simulink library "Collector_Unglazed"  (R2018b)
settings: Solver=ode45  StartTime=0.0  StopTime=10.0  RelTol=1e-3  EnableMultiTasking=on
undefined symbols (not defined in the file): Acol, path_carnot, Qdot, THBin, THBout
libraries: carnot x5
settings Model: Creator=bernd.hafner  LastModifiedBy=P41573
settings DataIOCC: LimitDataPoints=on  SaveFormat=Array  SignalLoggingSaveFormat=ModelDataLogs
settings OptimizationCC: ExpressionDepthLimit=2147483647  LifeSpan=inf
settings DebuggingCC: UnderspecifiedInitializationDetection=Classic  MergeDetectMultiDrivingBlocksExec=none  SolverPrmCheckMsg=warning  FcnCallInpInsideContextMsg=warning  StateNameClashWarn=warning  SFUnexpectedBacktrackingDiag=warning  SFNoUnconditionalDefaultTransitionDiag=warning  SFExecutionAtInitializationDiag=none
settings HardwareCC: ProdBitPerPointer=32  ProdBitPerSizeT=32  ProdBitPerPtrDiffT=32  ProdLargestAtomicFloat=None  ProdIntDivRoundTo=Undefined  ProdEndianess=Unspecified  ProdWordSize=32  ProdHWDeviceType=32-bit Generic
settings ModelReferenceCC: PropagateSignalLabelsOutOfModel=off
settings SFSimCC: SimUseLocalCustomCode=off
settings RTWCC: RTWUseLocalCustomCode=off
settings CodeAppCC: StateflowObjectComments=on
settings GRTTargetCC: TargetLangStandard=C89/C90 (ANSI)  GeneratePreprocessorConditionals=Disable all  CombineOutputUpdateFcns=off  GRTInterface=on
settings ConfigComp: CovMetricSettings=dw  CovHtmlReporting=on  CovSaveCumulativeToWorkspaceVar=on  CovSaveSingleToWorkspaceVar=on  CovExternalEMLEnable=off

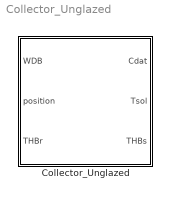
== system Collector_Unglazed ==
  Collector_Unglazed : Subsystem  mask(Unglazed solar thermal collector){tini=0.1, Ncollector=1, PathName=fullfile(path_carnot('libsl'), 'Source', 'Solar_Thermal', 'Collector_Unglazed', 'parameter_set'), FileName='DefaultCollectorUnglazed.mat', userPath=off, userParam=off, acol=2.544, len=2.1, nodes=10, fta=0.9, eps=0.9, u0l=40, u0c=1, u0g=40, u1l=8, u1c=1, u1g=8, u1e=0.01, hi=200, capa=5000, capf=4000, SensorTimeConstant=10, dplin=5504.4, dpqua=6222.096}
      mask prompts: tini "Initial temperature [°C]"; Ncollector "Number of collectors in parallel"; PathName "Path"; FileName "Parameter set"; userPath "Edit path and name of parameter set"; userParam "User defined parameters"; acol "Collector surface (aperture) in [m²]"; len "Length between inlet and outlet [m]"; nodes "Number of nodes (>=2)"; fta "Absorption coefficient of the absorber [-]"; eps "Thermal emissivity of the absorber (0..1)"; u0l "U0L heat transfer for losses [W/(m²*K)]"; u0c "U0C heat transfer for condensation [W/(m²*K)]"; u0g "U0G heat transfer for gains [W/(m²*K)]"; u1l "U1L wind dependent heat transfer for losses [W/(m²*K*m/s)]"; u1c "U1C wind dependent heat transfer for condensation [W/(m²*K*m/s)]"; u1g "U1G wind dependent heat transfer for gains [W/(m²*K*m/s)]"; u1e "U1E wind dependancy of optical efficiency in W/(m²*m/s)"; hi "HI heat transfer between collector and tube [W/(m²*K)]"; capa "Effective heat capacity of absorber [J/(m²*K)]"; capf "Effective heat capacity of fluid [J/(m²*K)]"; SensorTimeConstant "Time constant of temperature sensor [s]"; dplin "Linear pressure drop in Pa/(kg/s)"; dpqua "Quadratic pressure drop in Pa/(kg/s)²"
      mask help:
      | 2xN node model for an unglazed solar thermal collectors including condensation effects for temperatures below dewpoint.
      | c_abs*dTp/dt=qdot_solar-qdot_conv_gain-qdot_conv_loss-qdot_cond -qdot_sky-qdot_fluid
      | qdot_solar = absorbed_solar_radiation - U1E*Iglb*vwind
      | qdot_conv_gain = fconv * (U0G + U1G*vwind)*(Tp - Tamb)
      | qdot_conv_loss = (1-fconv)*(U0L + U1L*vwind)*(Tp - Tamb)
      | qdot_cond = fcond*(U0C + U1C*vwind)*ccond*(ps(Tdew) - ps(Tp))
      | qdot_sky = e * const_sigma*((Tp+273)^4 - (Tsky+273)^4)
      | qdot_fluid = HI*(Tp-Tfluid)
      | fconv = 1 if Tp > Tamb, 0 otherwise
      | fcond = 1 if Tp below dewpoint, 0 otherwise
      mask init:
      | [ok, param] = CarnotCallbacks_CollectorUnglazedConf('SetParameters',gcbh,PathName,FileName);
      mask Help: web(fullfile(path_carnot('help'),'Collector_Unglazed.html'),'-helpbrowser')
      mask TypeOptions tini: Collector_Unglazed/tini | T_Sensor1/t0
      mask TypeOptions Ncollector: Ncollector/Value | Gain/Gain | Gain3/Gain
      mask Callback userPath: [ok, param] = CarnotCallbacks_CollectorUnglazedConf('UserEdit',gcbh);
      mask Callback userParam: [ok, param] = CarnotCallbacks_CollectorUnglazedConf('UserEdit',gcbh);
      mask TypeOptions acol: Collector_Unglazed/acol
      mask TypeOptions len: Collector_Unglazed/len
      mask TypeOptions nodes: Collector_Unglazed/nodes
      mask TypeOptions fta: Collector_Unglazed/fta
      mask TypeOptions eps: Collector_Unglazed/e_sky
      mask TypeOptions u0l: Collector_Unglazed/uc0loss
      mask TypeOptions u0c: Collector_Unglazed/uc0
      mask TypeOptions u0g: Collector_Unglazed/uc0gain
      mask TypeOptions u1l: Collector_Unglazed/uc1loss
      mask TypeOptions u1c: Collector_Unglazed/uc1
      mask TypeOptions u1g: Collector_Unglazed/uc1gain
      mask TypeOptions u1e: Collector_Unglazed/uc1eta0
      mask TypeOptions hi: Collector_Unglazed/hi
      mask TypeOptions capa: Collector_Unglazed/c_abs
      mask TypeOptions capf: Collector_Unglazed/c_fl
      mask TypeOptions SensorTimeConstant: T_Sensor1/tc
      mask TypeOptions dplin: Collector_Unglazed/lin
      mask TypeOptions dpqua: Collector_Unglazed/qua
      mask DialogControl Container7 Prompt: Calculation
      mask DialogControl ParameterGroupVar Prompt: Picking a parameter set
      mask DialogControl Control3 Prompt: Carnot public data
      mask DialogControl Control3 Callback: [ok, file] = CarnotCallbacks_CollectorUnglazedConf('GetFilename',gcbh, 'public');
      mask DialogControl Control4 Prompt: Carnot internal data
      mask DialogControl Control4 Callback: [ok, file] = CarnotCallbacks_CollectorUnglazedConf('GetFilename',gcbh, 'internal');
      mask DialogControl Control2 Prompt: Selected path
      mask DialogControl Control2 Callback: [ok, file] = CarnotCallbacks_CollectorUnglazedConf('GetFilename',gcbh, 'selected');
      mask DialogControl Container9 Prompt: Parameter values
      mask DialogControl Container8 Prompt: Geometry
      mask DialogControl Container11 Prompt: Thermal
      mask DialogControl Container12 Prompt: Hydraulic
      mask DialogControl Control6 Prompt: Save in Carnot internal data
      mask DialogControl Control6 Callback: [ok, param] = CarnotCallbacks_CollectorUnglazedConf('SaveFilename',gcbh, 'internal','USTC');
      mask DialogControl Control5 Prompt: Save in selected path
      mask DialogControl Control5 Callback: [ok, param] = CarnotCallbacks_CollectorUnglazedConf('SaveFilename',gcbh, 'selected','USTC');
      mask Display:
      | % user defined picture file
      | picfile = fullfile(path_carnot('intlibsl'), ...
      |     'Source','Solar_Thermal','Collector_Unglazed','parameter_set', ...
      |      'Collector_CONF.jpg');
      | 
      | pic = false;
      | 
      | % show internal picture if defined
      | if ~BlockIsInCarnotLibrary    % if not located in library any more
      |     if exist(picfile)
      |         image(imread(picfile), [0.2, 0, 0.7, 1])
      |         set_param(gcb, 'BackgroundColor', 'White')
      |         pic = true;
      |     end
      | end
      | 
      | if ~pic % show public picture
      |     plot([0,70,70,0,0]/140+0.1,         [-0,-0,5,5,-0]/140+0.2, ...
      |         [30,30,100,100,30]/140+0.1,     [100,94,94,100,100]/140+0.2, ...
      |         [32,1]/140+0.1,                 [94,5]/140+0.2, ...
      |         [40,10]/140+0.1,                [94,5]/140+0.2, ...
      |         [49,19]/140+0.1,                [94,5]/140+0.2, ...
      |         [57,27]/140+0.1,                [94,5]/140+0.2, ...
      |         [65,35]/140+0.1,                [94,5]/140+0.2, ...
      |         [73,43]/140+0.1,                [94,5]/140+0.2, ...
      |         [82,51]/140+0.1,                [94,5]/140+0.2, ...
      |         [90,60]/140+0.1,                [94,5]/140+0.2,...
      |         [98,68]/140+0.1,                [94,5]/140+0.2)
      |     set_param(gcb, 'BackgroundColor', 'Yellow')
      | end

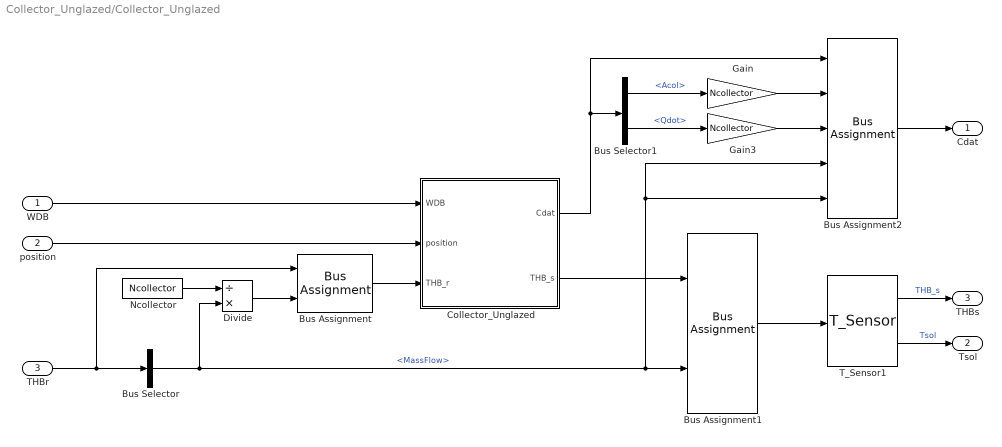
== system Collector_Unglazed/Collector_Unglazed ==
  WDB : Inport
  position : Inport  Port=2
  THBr : Inport  Port=3
  Bus Assignment : BusAssignment  AssignedSignals=MassFlow
  Bus Assignment1 : BusAssignment  AssignedSignals=MassFlow
  Bus Assignment2 : BusAssignment  AssignedSignals=Acol,Qdot,THBin.MassFlow,THBout.MassFlow
  Bus Selector : BusSelector  OutputSignals=MassFlow
  Bus Selector1 : BusSelector  OutputSignals=Acol,Qdot
  Collector_Unglazed : Subsystem  mask(Unglazed flat plate collector){acol=acol, len=len, fta=fta, e_sky=eps, uc0=u0c, uc1=u1c, uc0loss=u0l, uc1loss=u1l, uc0gain=u0g, uc1gain=u1g, uc1eta0=u1e, hi=hi, c_abs=capa, c_fl=capf, lin=dplin, qua=dpqua, tini=tini, nodes=nodes}
      mask prompts: acol "collector surface (aperture) in [m²]"; len "length between inlet and outlet [m]"; fta "absorption coefficient of the absorber [-]"; e_sky "e thermal emissivity of the absorber (0..1)"; uc0 "U0C heat transfer for condensation [W/(m²*K)]"; uc1 "U1C wind dependent heat transfer for condensation [W/(m²*K*m/s)]"; uc0loss "U0L heat transfer for losses [W/(m²*K)]"; uc1loss "U1L wind dependent heat transfer for losses [W/(m²*K*m/s)]"; uc0gain "U0G heat transfer for gains [W/(m²*K)]"; uc1gain "U1G wind dependent heat transfer for gains [W/(m²*K*m/s)]"; uc1eta0 "U1E wind dependancy of optical efficiency in W/(m²*m/s)"; hi "HI heat transfer between collector and tube [W/(m2.K)]"; c_abs "effective heat capacity of absorber [J/(m²*K)]"; c_fl "effective heat capacity of fluid [J/(m²*K)]"; lin "linear pressure drop in Pa/(kg/s)"; qua "quadratic pressure drop in Pa/(kg/s)²"; tini "initial temperature [degree centigrade]"; nodes "number of nodes (>=2)"
      mask help:
      | 2xN-nodes model:
      | c_abs*dTp/dt=qdot_solar-qdot_conv_gain-qdot_conv_loss-qdot_cond
      |             -qdot_sky-qdot_fluid
      | qdot_solar = absorbed_solar_radiation - U1E*Iglb*vwind
      | qdot_conv_gain = fconv * (U0G + U1G*vwind)*(Tp - Tamb)
      | qdot_conv_loss = (1-fconv)*(U0L + U1L*vwind)*(Tp - Tamb)
      | qdot_cond = fcond*(U0C + U1C*vwind)*ccond*(ps(Tdew) - ps(Tp))
      | qdot_sky = e * const_sigma*(Tp^4 - Tsky^4)
      | qdot_fluid = HI*(Tp-Tfluid)
      | fconv = 1 if Tp > Tamb, 0 otherwise
      | fcond = 1 if Tp below dewpoint, 0 otherwise
      | Look under mask to change the incidence angle modifier, the pressure drop and the radiation calculation method.
      mask init:
      | acol = max(acol, 0.01);
      | fta = max(fta,0);
      | inv_c_abs = 1/max(c_abs,1);
      | inv_c_fl = 1/max(c_fl,1);
      mask Help: web(fullfile(path_carnot('help'),'Collector_Unglazed.html'),'-helpbrowser')
      mask DialogControl ParameterTabVar0 Prompt: Geometry
      mask DialogControl ParameterTabVar01 Prompt: Coll.Parameters
      mask DialogControl ParameterTabVar012 Prompt: Hydraulic
      mask DialogControl ParameterTabVar0123 Prompt: Calculation
      mask Display: plot(-30,-30,130,120,[0,70,70,0,0],[-0,-0,5,5,-0],[30,30,100,100,30],[100,94,94,100,100],[32,1],[94,5],[40,10],[94,5],[49,19],[94,5],[57,27],[94,5],[65,35],[94,5],[73,43],[94,5],[82,51],[94,5],[90,60],[94,5],[98,68],[94,5])
  Divide : Product  Inputs=/*
  Gain : Gain  Gain=Ncollector
  Gain3 : Gain  Gain=Ncollector
  Ncollector : Constant  Value=Ncollector
  T_Sensor1 : carnot/Control/T_Sensor  tc=SensorTimeConstant  t0=tini
      settings: SourceProductName=Carnot
  Cdat : Outport
  Tsol : Outport  Port=2
  THBs : Outport  Port=3
  wires:
  Bus Assignment2/1 -> Cdat/1
  Gain3/1 -> Bus Assignment2/3
  Gain/1 -> Bus Assignment2/2
  Bus Selector1/2 -> Gain3/1  "<Qdot>"
  Bus Selector1/1 -> Gain/1  "<Acol>"
  Divide/1 -> Bus Assignment/2
  Ncollector/1 -> Divide/1
  Bus Selector/1 -> Bus Assignment1/2, Bus Assignment2/4, Bus Assignment2/5, Divide/2  "<MassFlow>"
  Bus Assignment1/1 -> T_Sensor1/1
  Bus Assignment/1 -> Collector_Unglazed/3(THB_r)
  Collector_Unglazed/1(Cdat) -> Bus Selector1/1, Bus Assignment2/1
  THBr/1 -> Bus Selector/1, Bus Assignment/1
  position/1 -> Collector_Unglazed/2(position)
  WDB/1 -> Collector_Unglazed/1(WDB)
  Collector_Unglazed/2(THB_s) -> Bus Assignment1/1
  T_Sensor1/1 -> THBs/1  "THB_s"
  T_Sensor1/2 -> Tsol/1  "Tsol"

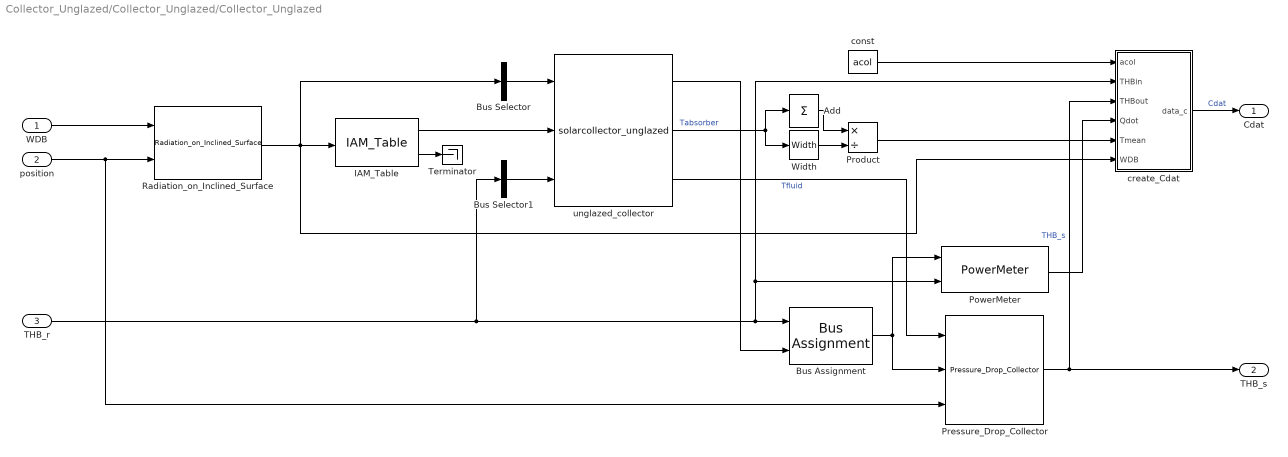
== system Collector_Unglazed/Collector_Unglazed/Collector_Unglazed ==
  WDB : Inport
  position : Inport  Port=2
  THB_r : Inport  Port=3
  Add : Sum  Inputs=1
  Bus Assignment : BusAssignment  AssignedSignals=Temperature
  Bus Selector : BusSelector  OutputSignals=Solar_Radiation_direct_surface,Solar_Radiation_diffuse_surface,Temperature_Ambient,Temperature_Sky_Radiation,Relative_Humidity,Station_Pressure,Wind_Speed  OutputAsBus=on
  Bus Selector1 : BusSelector  OutputSignals=Temperature,MassFlow,Pressure,FluidType,FluidMix  OutputAsBus=on
  IAM_Table : carnot/Source/Solar_Thermal/IncidenceAngleModifier/IAM_Table  fta=fta  angle=[0:5:90]  Kb="[1.0000    1.0000    0.9999    0.9996    0.9991    0.9982    0.9965  0.9935    0.9886    0.9807    0.9678    0.9473    0.9148    0.8638   0.7846    0.6644    0.4907    0.2599    0.0000]"  Kd=0.92
      settings: SourceProductName=Carnot
  PowerMeter : carnot/Control/PowerMeter
      settings: SourceProductName=Carnot
  Pressure_Drop_Collector : carnot/Basic/Pressure_Drop/Pressure_Drop_Collector  len=len  lin=lin  qua=qua
      settings: SourceProductName=Carnot
  Product : Product  Inputs=*/  RndMeth=Zero
  Radiation_on_Inclined_Surface : carnot/Weather/Radiation_on_Inclined_Surface  sky=Perez 1990  reflect=0.2
      settings: SourceProductName=Carnot
  Terminator : Terminator
  Width : Width
  const : Constant  Value=acol
  create_Cdat : Subsystem
  unglazed_collector : S-Function  FunctionName=solarcollector_unglazed  Parameters=acol, uc0, uc1, uc0loss, uc1loss, uc0gain, uc1gain, e_sky, uc1eta0, hi, inv_c_abs, inv_c_fl, len, tini, nodes  SFunctionDeploymentMode=off  EnableBusSupport=off
  Cdat : Outport
  THB_s : Outport  Port=2
  wires:
  unglazed_collector/3 -> Pressure_Drop_Collector/1  "Tfluid"
  Pressure_Drop_Collector/1 -> THB_s/1, create_Cdat/3(THBout)  "THB_s"
  Width/1 -> Product/2
  Product/1 -> create_Cdat/5(Tmean)
  Add/1 -> Product/1
  PowerMeter/1 -> create_Cdat/4(Qdot)
  create_Cdat/1(data_c) -> Cdat/1  "Cdat"
  const/1 -> create_Cdat/1(acol)
  unglazed_collector/2 -> Width/1, Add/1  "Tabsorber"
  unglazed_collector/1 -> Bus Assignment/2
  IAM_Table/2 -> Terminator/1
  Bus Selector1/1 -> unglazed_collector/3
  Bus Selector/1 -> unglazed_collector/1
  THB_r/1 -> PowerMeter/2, create_Cdat/2(THBin), Bus Assignment/1, Bus Selector1/1
  WDB/1 -> Radiation_on_Inclined_Surface/1
  position/1 -> Radiation_on_Inclined_Surface/2, Pressure_Drop_Collector/3
  Radiation_on_Inclined_Surface/1 -> IAM_Table/1, Bus Selector/1, create_Cdat/6(WDB)
  Bus Assignment/1 -> PowerMeter/1, Pressure_Drop_Collector/2
  IAM_Table/1 -> unglazed_collector/2

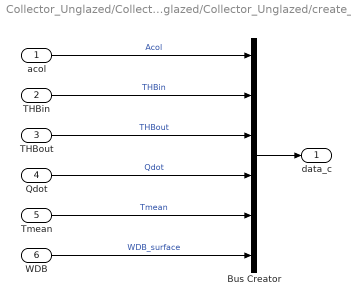
== system Collector_Unglazed/Collector_Unglazed/Collector_Unglazed/create_Cdat ==
  acol : Inport
  THBin : Inport  Port=2
  THBout : Inport  Port=3
  Qdot : Inport  Port=4
  Tmean : Inport  Port=5
  WDB : Inport  Port=6
  Bus Creator : BusCreator  Inputs=6
  data_c : Outport
  wires:
  Tmean/1 -> Bus Creator/5  "Tmean"
  Qdot/1 -> Bus Creator/4  "Qdot"
  Bus Creator/1 -> data_c/1
  WDB/1 -> Bus Creator/6  "WDB_surface"
  THBout/1 -> Bus Creator/3  "THBout"
  THBin/1 -> Bus Creator/2  "THBin"
  acol/1 -> Bus Creator/1  "Acol"
